simulink model "bloco_simulacao2"  (R2021a)
settings: Solver=VariableStepAuto  StartTime=0.0  StopTime=10.0  RelTol=1e-3
values from neighbouring files (symbols this model uses):
  B = 0    [P1_script.m]    (also in simulacao1.m)
  J = 0.001    [P1_script.m]    (also in simulacao1.m = 0.00252)
  La = 1.7e-3    (= 0.0017)    [P1_script.m]    (also in simulacao1.m)
  Ra = 0.26    [P1_script.m]    (also in simulacao1.m)
undefined symbols (not defined in the file or in its folder): K
libraries: ee_lib x1
settings Model: Creator=taylo  LastModifiedBy=taylo

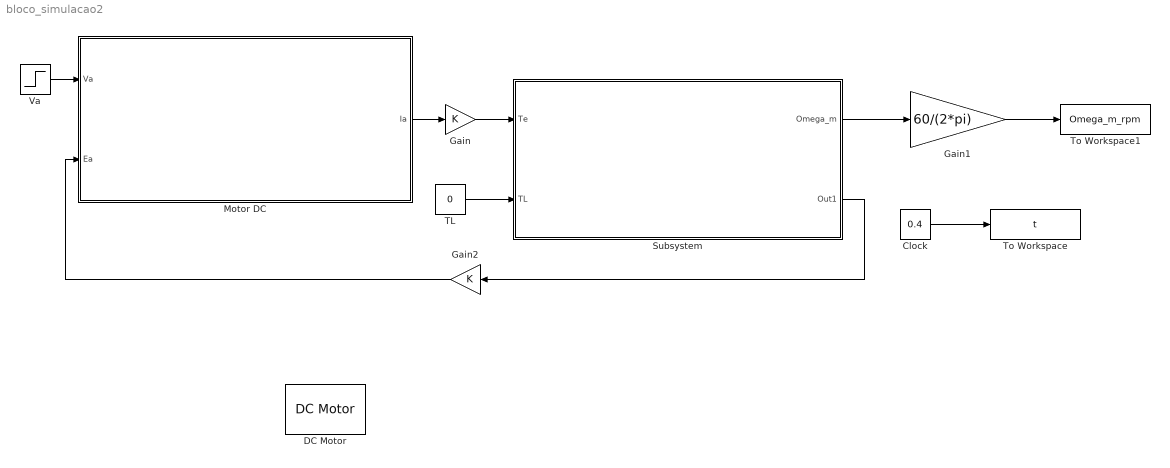
== system bloco_simulacao2 ==
  Clock : Constant  Value=0.4
  DC Motor : ee_lib/Electromechanical/Brushed Motors/DC Motor  field_option=ee.enum.field_option.pm  Rf=100 Ohm  Lf=1 H  Laf=0.15 H  If0=0 A  parameterization=ee.enum.dcparam_option.circuit_param  Ra=3.9 Ohm  La=12e-6 H  emf_or_torque=ee.enum.emf_or_torque.kv  Kv=0.072e-3 V/rpm  Ki=6.876e-4 N*m/A  T_stall=0.24e-3 N*m  w_max=19100 rpm  w_rated=15000 rpm  P_rated=0.08 W  V_rated=1.5 V  J=0.01 g*cm^2  lam_param=ee.enum.lam_param.damping  lam=0 N*m/(rad/s)  i_noload=0 A  V_i_noload=1.5 V  speed0=0 rpm  enable_fault_armature=ee.enum.faults.faultEnable.no  rev_faulted=1 / 3  G_faulted_armature=1e-5 S  fault_trigger_armature=ee.enum.faults.faultTrigger.temporal  t_fault_armature=1 s  max_permissible_current_armature=inf A  t_fail_on_current_armature=1 s  enable_fault_field=ee.enum.faults.faultEnable.no  G_faulted_field=1e-5 S  fault_trigger_field=ee.enum.faults.faultTrigger.temporal  t_fault_field=1 s  max_permissible_current_field=inf A  t_fail_on_current_field=1 s  fault_action=ee.enum.faults.faultAction.none  alpha=3.93e-3 1/K  Tmeas=25 degC  thermal_mass=100 J/K  initial_temperature=25 degC
  Gain : Gain  Gain=K
  Gain1 : Gain  Gain=60/(2*pi)
  Gain2 : Gain  Gain=K
  Motor DC : Subsystem
  Subsystem : Subsystem
  TL : Constant  Value=0
  To Workspace : ToWorkspace  VariableName=t  SaveFormat=Timeseries  SampleTime=-1
  To Workspace1 : ToWorkspace  VariableName=Omega_m_rpm  SaveFormat=Timeseries  SampleTime=-1
  Va : Step  After=70  SampleTime=0
  wires:
  Motor DC/1(Ia) -> Gain/1
  Gain/1 -> Subsystem/1(Te)
  TL/1 -> Subsystem/2(TL)
  Va/1 -> Motor DC/1(Va)
  Subsystem/1(Omega_m) -> Gain1/1
  Subsystem/2(Out1) -> Gain2/1
  Gain2/1 -> Motor DC/2(Ea)
  Clock/1 -> To Workspace/1
  Gain1/1 -> To Workspace1/1

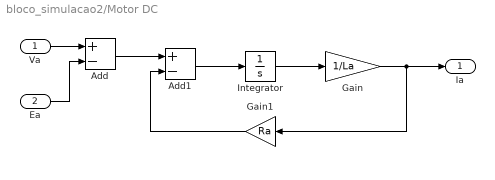
== system bloco_simulacao2/Motor DC ==
  Va : Inport
  Ea : Inport  Port=2
  Add : Sum  Inputs=+-
  Add1 : Sum  Inputs=+-
  Gain : Gain  Gain=1/La
  Gain1 : Gain  Gain=Ra
  Integrator : Integrator
  Ia : Outport
  wires:
  Add1/1 -> Integrator/1
  Gain1/1 -> Add1/2
  Add/1 -> Add1/1
  Va/1 -> Add/1
  Integrator/1 -> Gain/1
  Ea/1 -> Add/2
  Gain/1 -> Gain1/1, Ia/1

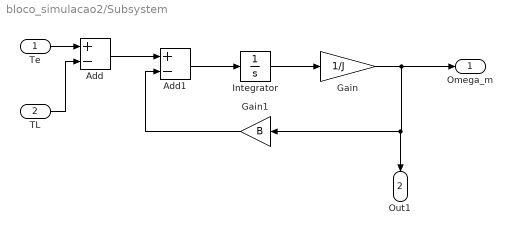
== system bloco_simulacao2/Subsystem ==
  Te : Inport
  TL : Inport  Port=2
  Add : Sum  Inputs=+-
  Add1 : Sum  Inputs=+-
  Gain : Gain  Gain=1/J
  Gain1 : Gain  Gain=B
  Integrator : Integrator
  Omega_m : Outport
  Out1 : Outport  Port=2
  wires:
  Te/1 -> Add/1
  Gain/1 -> Omega_m/1, Out1/1, Gain1/1
  Add/1 -> Add1/1
  TL/1 -> Add/2
  Add1/1 -> Integrator/1
  Gain1/1 -> Add1/2
  Integrator/1 -> Gain/1
